simulink model "ErdeMond"  (Simulink 7.1)
settings: Solver=ode23tb  StartTime=0.0  StopTime=2300000  RelTol=1e-3
libraries: simulink x2
settings Model: Creator=Meisel  LastModifiedBy=Meisel

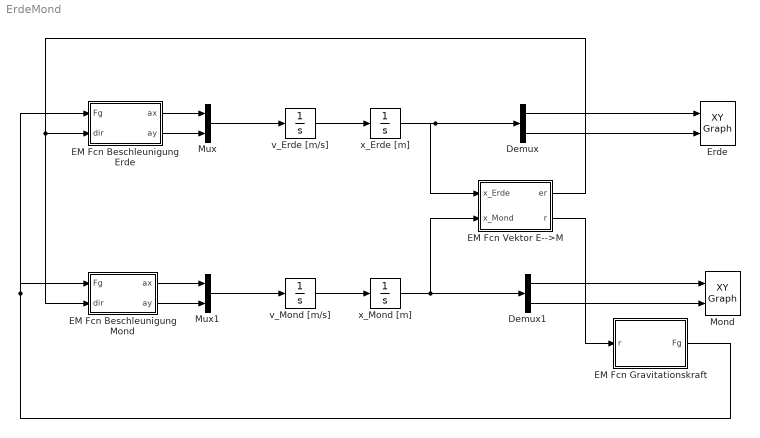
== system ErdeMond ==
  Demux : Demux  Outputs=2
  Demux1 : Demux  Outputs=2
  EM Fcn Beschleunigung Erde : Stateflow chart
  EM Fcn Beschleunigung Mond : Stateflow chart
  EM Fcn Gravitationskraft : Stateflow chart
  EM Fcn Vektor E-->M : Stateflow chart
  Erde : simulink/Sinks/XY Graph  SystemSampleTime=-1  xmin=-0.2*10^8  xmax=0.2*10^8  ymin=-0.2*10^8  ymax=0.2*10^8  st=-1
  Mond : simulink/Sinks/XY Graph  SystemSampleTime=-1  xmin=-0.5*10^9  xmax=0.5*10^9  ymin=-0.5*10^9  ymax=0.5*10^9  st=-1
  Mux : Mux  Inputs=2
  Mux1 : Mux  Inputs=2
  v_Erde [m/s] : Integrator  InitialCondition=[0,-12.40]
  v_Mond [m/s] : Integrator  InitialCondition=[0,1000]  IgnoreLimit=on
  x_Erde [m] : Integrator  InitialCondition=[0,0]
  x_Mond [m] : Integrator  InitialCondition=[-380*10^6,0]
  wires:
  v_Erde [m/s]/1 -> x_Erde [m]/1
  Mux/1 -> v_Erde [m/s]/1
  x_Erde [m]/1 -> Demux/1, EM Fcn Vektor E-->M/1(x_Erde)
  Demux/1 -> Erde/1
  Demux/2 -> Erde/2
  v_Mond [m/s]/1 -> x_Mond [m]/1
  Mux1/1 -> v_Mond [m/s]/1
  x_Mond [m]/1 -> Demux1/1, EM Fcn Vektor E-->M/2(x_Mond)
  Demux1/1 -> Mond/1
  Demux1/2 -> Mond/2
  EM Fcn Beschleunigung Erde/1(ax) -> Mux/1
  EM Fcn Beschleunigung Erde/2(ay) -> Mux/2
  EM Fcn Beschleunigung Mond/1(ax) -> Mux1/1
  EM Fcn Beschleunigung Mond/2(ay) -> Mux1/2
  EM Fcn Gravitationskraft/1(Fg) -> EM Fcn Beschleunigung Mond/1(Fg), EM Fcn Beschleunigung Erde/1(Fg)
  EM Fcn Vektor E-->M/1(er) -> EM Fcn Beschleunigung Erde/2(dir), EM Fcn Beschleunigung Mond/2(dir)
  EM Fcn Vektor E-->M/2(r) -> EM Fcn Gravitationskraft/1(r)

== matlab function EM Fcn Beschleunigung Erde ==
  data: Fg input double; ax output double; ay output double; dir input double
function [ax,ay] = AccE(Fg,dir)
% Embedded MATLAB 
% Fg : Gravitationskraft
% dir : Einheitsvektor E-->M

m_Erde=5.9*10^24;

ax = Fg/m_Erde*dir(1);
ay = Fg/m_Erde*dir(2);

== matlab function EM Fcn Gravitationskraft ==
  data: r input double; Fg output double
function Fg = Grav(r)
% Embedded MATLAB

G=66.7*10^-12;
m_Erde=5.9*10^24;
m_Mond=7.3*10^22;

Fg=G*m_Erde*m_Mond/(r*r);

== matlab function EM Fcn Beschleunigung Mond ==
  data: Fg input double; ax output double; ay output double; dir input double
function [ax,ay] = AccM(Fg,dir)
% Fg : Gravitationskraft
% dir : Einheitsvektor E-->M


m_Mond=7.3*10^22;

ax = -Fg/m_Mond*dir(1);
ay = -Fg/m_Mond*dir(2);

== matlab function EM Fcn Vektor E-->M ==
  data: er output double; x_Erde input double; r output double; x_Mond input double
function [er, r] = AbstDir(x_Erde, x_Mond)
% Embedded MATLAB

rVek = x_Mond-x_Erde;
er   = rVek/norm(rVek);  % Einheitsvektor E-->M
r    = norm(rVek);       % Abstand E-->M
